simulink model "scheme"  (R2025b)
settings: Solver=ode5  StartTime=0.0  StopTime=100  FixedStep=1e-3  RelTol=1e-6  EnableMultiTasking=on
settings Model: ExtModeTrigDuration=100000  Creator=lab  LastModifiedBy=lucag
settings SolverCC: AlgebraicLoopSolver=TrustRegion
settings DataIOCC: SaveFormat=Array  SignalLoggingSaveFormat=ModelDataLogs  ReturnWorkspaceOutputs=off
settings OptimizationCC: ExpressionDepthLimit=2147483647.0
settings DebuggingCC: UnderspecifiedInitializationDetection=Classic  MergeDetectMultiDrivingBlocksExec=none  SolverPrmCheckMsg=warning  FcnCallInpInsideContextMsg=warning  UnconnectedInputMsg=warning  UnconnectedOutputMsg=warning  UnconnectedLineMsg=warning  StateNameClashWarn=warning  SFUnexpectedBacktrackingDiag=warning  SFNoUnconditionalDefaultTransitionDiag=warning  SFExecutionAtInitializationDiag=none  ArithmeticOperatorsInVariantConditions=warning
settings HardwareCC: ProdBitPerLong=64.0  ProdHWDeviceType=Intel->x86-64 (Linux 64)
settings ModelReferenceCC: EnableRefExpFcnMdlSchedulingChecks=on  PropagateSignalLabelsOutOfModel=off
settings SFSimCC: SimUseLocalCustomCode=off  SimParseCustomCode=off  CustomCodeUndefinedFunction=UseInterfaceOnly
settings RTWCC: SystemTargetFile=sldrt.tlc  TemplateMakefile=sldrt.tmf  RTWUseLocalCustomCode=off  RTWCompilerOptimization=on  GPUComputeCapability=3.5  DLArmComputeVersion=19.05  Description=Simulink Desktop Real-Time
settings CodeAppCC: MaxIdLength=95.0  StateflowObjectComments=on
settings STFCustomTargetCC: SystemTargetFile=sldrt.tlc  TargetLangStandard=C99 (ISO)  ModelReferenceCompliant=off  ConcurrentExecutionCompliant=off  MATLABClassNameForMDSCustomization=Simulink.SoftwareTarget.TargetSpecificTriggerConfigurationBase
settings SimulinkDesktopRealTimeCC: TargetLibSuffix=_sldrt.a  SupportVariableSizeSignals=off  TargetLangStandard=C89/C90 (ANSI)  MultiwordLength=2048.0  DynamicStringBufferSize=256.0  PreserveMATLABNamespacesInGeneratedCode=on  ExtModeStaticAllocSize=1000000.0  ExtModeTransport=0.0  ParMdlRefBuildCompliant=on  TargetPreCompLibLocation=C:\Program Files\MATLAB\R2025b\toolbox\sldrt\lib\win64  SubcomponentCodeInterfacePackaging=Reusable function
settings ConfigComp: CovMetricSettings=dw  CovSaveCumulativeToWorkspaceVar=on  CovSaveSingleToWorkspaceVar=on  CovExternalEMLEnable=off  CovSFcnEnable=off

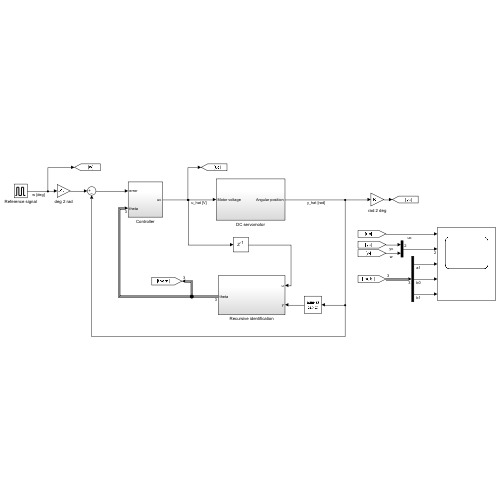
[thumbnail: Simulink's stored preview of the top-level diagram]
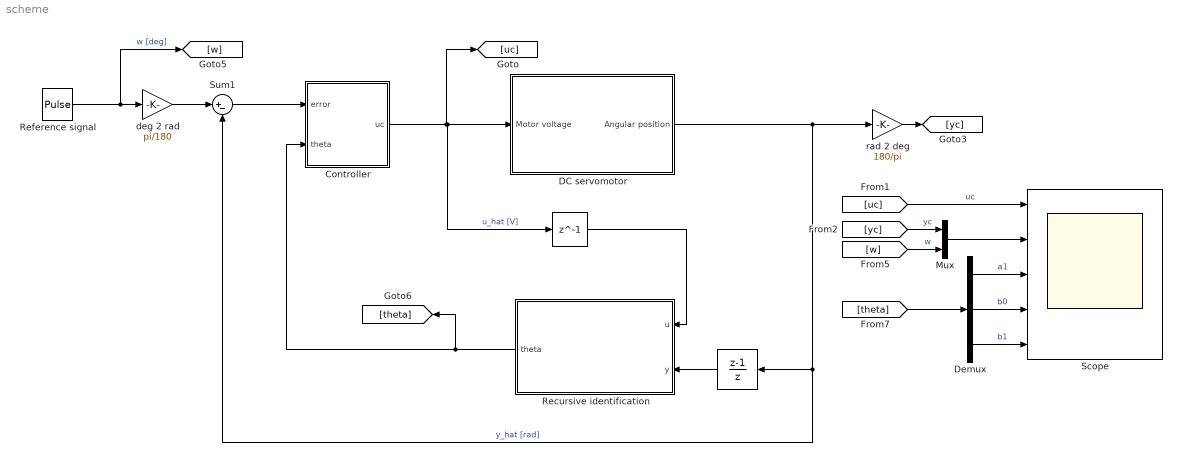
== system scheme ==
  " " : Delay  DelayLength=1  InitialCondition=0
  "  " : DiscreteTransferFcn  Numerator=[1 -1]  Denominator=[1 0]
  Controller : Subsystem
  DC servomotor : Subsystem
  Demux : Demux  Outputs=3
  Mux : Mux  Inputs=2
  Recursive identification : Subsystem
  "Reference signal " : DiscretePulseGenerator  PulseType=Time based  Amplitude=100  Period=5  PulseWidth=50
  Scope : Scope  NumInputPorts=5
      settings: TimeSpan=10  ActiveDisplayString=5  ActiveDisplayYMinimum=-0.76531009768731917  ActiveDisplayYMaximum=1.102580655761314  DataLoggingVariableName=sim_res
  Sum1 : Sum  Inputs=|+-
  deg 2 rad : Gain  Gain=pi/180
  rad 2 deg : Gain  Gain=180/pi
  wires:
  [uc] -> Scope/1  "uc"
  [yc] -> Mux/1  "yc"
  [w] -> Mux/2  "w"
  Mux/1 -> Scope/2
  Demux/1 -> Scope/3  "a1"
  Demux/2 -> Scope/4  "b0"
  Demux/3 -> Scope/5  "b1"
  [theta] -> Demux/1
  " "/1 -> Recursive identification/1(u)
  rad 2 deg/1 -> [yc]
  deg 2 rad/1 -> Sum1/1
  DC servomotor/1(Angular position) -> Sum1/2, "  "/1, rad 2 deg/1  "y_hat [rad]"
  "  "/1 -> Recursive identification/2(y)
  Recursive identification/1("theta ") -> [theta], Controller/2(theta)
  Controller/1(uc) -> DC servomotor/1("Motor voltage "), " "/1, [uc]  "u_hat [V]"
  Sum1/1 -> Controller/1(error)
  "Reference signal "/1 -> [w], deg 2 rad/1  "w [deg]"

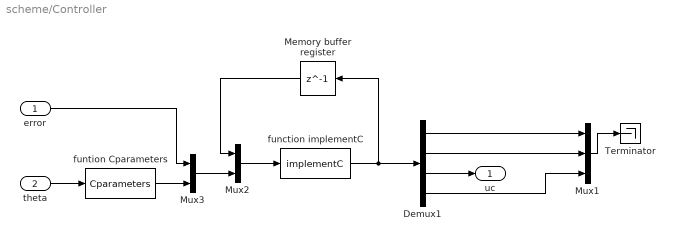
== system scheme/Controller ==
  error : Inport
  theta : Inport  Port=2
  Demux1 : Demux
  Memory buffer register : Delay  DelayLength=1  InitialCondition=[0 0 0 0]'
  Mux1 : Mux  Inputs=3
  Mux2 : Mux  Inputs=2
  Mux3 : Mux  Inputs=2
  Terminator : Terminator
  function implementC : MATLABFcn  MATLABFcn=implementC
  funtion Cparameters : MATLABFcn  MATLABFcn=Cparameters
  uc : Outport
  wires:
  theta/1 -> funtion Cparameters/1
  error/1 -> Mux3/1
  function implementC/1 -> Memory buffer register/1, Demux1/1
  Memory buffer register/1 -> Mux2/1
  Mux2/1 -> function implementC/1
  funtion Cparameters/1 -> Mux3/2
  Demux1/3 -> uc/1
  Mux3/1 -> Mux2/2
  Mux1/1 -> Terminator/1
  Demux1/1 -> Mux1/1
  Demux1/2 -> Mux1/2
  Demux1/4 -> Mux1/3

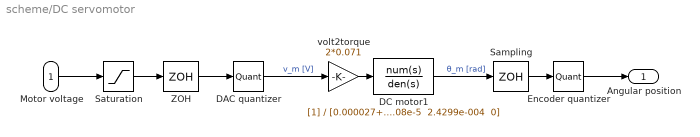
== system scheme/DC servomotor ==
  "Motor voltage " : Inport
  DAC quantizer : Quantizer  QuantizationInterval=10/2^13
  DC motor1 : TransferFcn  Denominator="[0.000027+1.08e-5  2.4299e-004  0]"
  Encoder quantizer : Quantizer  QuantizationInterval=2*pi/3000
  Sampling : ZeroOrderHold  SampleTime=0.001
  Saturation : Saturate  UpperLimit=3  LowerLimit=-3
  ZOH : ZeroOrderHold  SampleTime=0.001
  volt2torque : Gain  Gain=2*0.071
  Angular position : Outport
  wires:
  Sampling/1 -> Encoder quantizer/1
  Saturation/1 -> ZOH/1
  ZOH/1 -> DAC quantizer/1
  "Motor voltage "/1 -> Saturation/1
  DAC quantizer/1 -> volt2torque/1  "v_m [V]"
  Encoder quantizer/1 -> Angular position/1
  DC motor1/1 -> Sampling/1  "θ_m [rad]"
  volt2torque/1 -> DC motor1/1

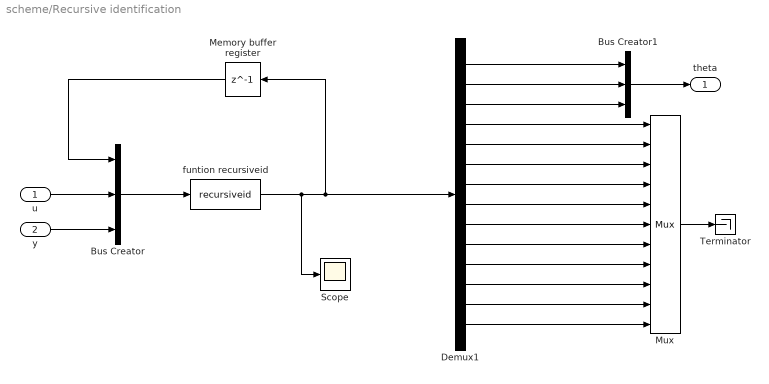
== system scheme/Recursive identification ==
  u : Inport
  y : Inport  Port=2
  Bus Creator : BusCreator  Inputs=3
  Bus Creator1 : BusCreator  Inputs=3
  Demux1 : Demux  Outputs=14
  Memory buffer register : Delay  DelayLength=1  InitialCondition=[-0.2 0.02 0.001 0 0 reshape(0.01*eye(3),9,1)']'
  Mux : Mux  Inputs=11
  Scope : Scope
      settings: ActiveDisplayYMinimum=-1  ActiveDisplayYMaximum=1
  Terminator : Terminator
  funtion recursiveid : MATLABFcn  MATLABFcn=recursiveid
  "theta " : Outport  PortDimensions=3
  wires:
  Bus Creator/1 -> funtion recursiveid/1
  Demux1/3 -> Bus Creator1/3
  Demux1/1 -> Bus Creator1/1
  Demux1/2 -> Bus Creator1/2
  funtion recursiveid/1 -> Scope/1, Memory buffer register/1, Demux1/1
  Bus Creator1/1 -> "theta "/1
  y/1 -> Bus Creator/3
  u/1 -> Bus Creator/2
  Memory buffer register/1 -> Bus Creator/1
  Demux1/4 -> Mux/1
  Demux1/5 -> Mux/2
  Demux1/6 -> Mux/3
  Demux1/7 -> Mux/4
  Demux1/8 -> Mux/5
  Demux1/9 -> Mux/6
  Demux1/10 -> Mux/7
  Demux1/11 -> Mux/8
  Demux1/12 -> Mux/9
  Demux1/13 -> Mux/10
  Demux1/14 -> Mux/11
  Mux/1 -> Terminator/1
